simulink library "Collector_EN12975_FlatPlate_CONF"  (R2016b)
settings: Solver=ode45  StartTime=0.0  StopTime=10.0  RelTol=1e-3  EnableMultiTasking=on
undefined symbols (not defined in the file): Acol, path_carnot, Qdot, THBin, THBout
libraries: carnot x2
settings Model: Creator=lena.frank  LastModifiedBy=drhf
settings DataIOCC: LimitDataPoints=on  SaveFormat=Array  SignalLoggingSaveFormat=ModelDataLogs
settings OptimizationCC: ExpressionDepthLimit=2147483647  LifeSpan=inf
settings DebuggingCC: UnderspecifiedInitializationDetection=Classic  MergeDetectMultiDrivingBlocksExec=none  SolverPrmCheckMsg=warning  FcnCallInpInsideContextMsg=warning  StateNameClashWarn=warning  SFUnexpectedBacktrackingDiag=warning  SFNoUnconditionalDefaultTransitionDiag=warning  SFExecutionAtInitializationDiag=none
settings HardwareCC: ProdBitPerPointer=32  ProdBitPerSizeT=32  ProdBitPerPtrDiffT=32  ProdLargestAtomicFloat=None  ProdIntDivRoundTo=Undefined  ProdEndianess=Unspecified  ProdWordSize=32  ProdHWDeviceType=32-bit Generic
settings ModelReferenceCC: PropagateSignalLabelsOutOfModel=off
settings GRTTargetCC: TargetLangStandard=C89/C90 (ANSI)  GeneratePreprocessorConditionals=Disable all  CombineOutputUpdateFcns=off  GRTInterface=on
settings ConfigComp: CovMetricSettings=dw  CovHtmlReporting=on  CovSaveCumulativeToWorkspaceVar=on  CovSaveSingleToWorkspaceVar=on  CovExternalEMLEnable=off

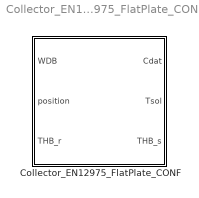
== system Collector_EN12975_FlatPlate_CONF ==
  Collector_EN12975_FlatPlate_CONF : Subsystem  mask(configurated Flat Plate Solar Thermal Collector){tini=20, Ncollector=2, PathName=fullfile(path_carnot('libsl'), 'Source','Solar_Thermal','Collector_EN12975_FlatPlate_CONF','parameter_set'), FileName='DefaultCollectorFlatPlate.mat', userPath=off, userParam=off, acol=2.5, len=2.3, fta=0.75, c1=3.5, c2=0.01, c3=0, c4=0, c5=7000, c6=0, b0=0.1, Kd=0.92, dplin=10, dpqua=10, SensorTimeConstant=10}
      mask prompts: tini "initial temperature [°C]"; Ncollector "Number of collectors in parallel"; PathName "Path"; FileName "Parameter set"; userPath "Edit path and name of parameter set"; userParam "User defined parameters"; acol "A : collector surface  [m²]"; len "length between inlet and outlet [m]"; fta "F'(TauAlfa)"; c1 "c1 : heat loss coefficient at (Tm-Ta)=0  [W/(m²*K)]"; c2 "c2: temperature dependence of the heat loss coefficient [W/(m*K)²]"; c3 "c3 : wind speed dependence of the heat loss coefficient [J/(m³K)]"; c4 "c4 : sky temperature dependence of the heat loss coefficient [W/(m²K)]"; c5 "c5 : effective thermal capacity [J/(m²K)]"; c6 "c6 : wind dependence of conversion factor [s/m]"; b0 "b0 : constant for the calculation of the incident angle modifier (direct radiation)"; Kd "Kd : Incidence angle modifier diffuse radiation"; dplin "linear pressure drop in Pa/(kg/s)"; dpqua "quadratic pressure drop in Pa/(kg/s)²"; SensorTimeConstant "time constant of sensor [s]"
      mask help:
      | Dynamic 1-node collector model according to EN 12975 standard using the b0 model for flat plate collector optics.
      | This block uses predefined parameter sets.
      mask init:
      | % callback to set parameters of model
      | [ok, param] = CarnotCallbacks_CollectorEN12975FlatPlateConf('SetParameters',gcbh,PathName,FileName);
      mask Help: web(fullfile(path_carnot('help'),'collector_en12975.html'),'-helpbrowser')
      mask TypeOptions tini: Collector_EN12975_FlatPlate/tini | T_Sensor1/t0
      mask TypeOptions Ncollector: Ncollector/Value
      mask Callback userPath: [ok, param] = CarnotCallbacks_CollectorEN12975FlatPlateConf('UserEdit',gcbh);
      mask Callback userParam: [ok, param] = CarnotCallbacks_CollectorEN12975FlatPlateConf('UserEdit',gcbh);
      mask TypeOptions acol: Collector_EN12975_FlatPlate/acol
      mask TypeOptions len: Collector_EN12975_FlatPlate/len
      mask TypeOptions fta: Collector_EN12975_FlatPlate/fta
      mask TypeOptions c1: Collector_EN12975_FlatPlate/c1
      mask TypeOptions c2: Collector_EN12975_FlatPlate/c2
      mask TypeOptions c3: Collector_EN12975_FlatPlate/c3
      mask TypeOptions c4: Collector_EN12975_FlatPlate/c4
      mask TypeOptions c5: Collector_EN12975_FlatPlate/c5
      mask TypeOptions c6: Collector_EN12975_FlatPlate/c6
      mask TypeOptions b0: Collector_EN12975_FlatPlate/b0
      mask TypeOptions Kd: Collector_EN12975_FlatPlate/Kd
      mask TypeOptions dplin: Collector_EN12975_FlatPlate/lin
      mask TypeOptions dpqua: Collector_EN12975_FlatPlate/qua
      mask TypeOptions SensorTimeConstant: T_Sensor1/tc
      mask DialogControl Control3 Prompt: Carnot public data
      mask DialogControl Control3 Callback: [ok, file] = CarnotCallbacks_CollectorEN12975FlatPlateConf('GetFilename',gcbh,'public');
      mask DialogControl Control4 Prompt: Carnot internal data
      mask DialogControl Control4 Callback: [ok, file] = CarnotCallbacks_CollectorEN12975FlatPlateConf('GetFilename',gcbh,'internal');
      mask DialogControl Control5 Prompt: Selected path
      mask DialogControl Control5 Callback: [ok, file] = CarnotCallbacks_CollectorEN12975FlatPlateConf('GetFilename',gcbh,'selected');
      mask DialogControl Control6 Prompt: Save in Carnot internal data
      mask DialogControl Control6 Callback: [ok, param] = CarnotCallbacks_CollectorEN12975FlatPlateConf('SaveFilename',gcbh,'internal','FPC');
      mask DialogControl Control7 Prompt: Save in selected path
      mask DialogControl Control7 Callback: [ok, param] = CarnotCallbacks_CollectorEN12975FlatPlateConf('SaveFilename',gcbh,'selected','FPC');
      mask Display:
      | % user defined picture file
      | picfile = fullfile(path_carnot('intlibsl'), ...
      |     'Source','Solar_Thermal','Collector_EN12975_FlatPlate_CONF','parameter_set', ...
      |     'Collector_CONF.jpg');
      | 
      | pic = false;
      | 
      | % show internal picture if defined
      | if ~BlockIsInCarnotLibrary    % if not located in library any more
      |     if exist(picfile)
      |         image(imread(picfile), [0.2, 0, 0.6, 1])
      |         set_param(gcb, 'BackgroundColor', 'White')
      |         pic = true;
      |     end
      | end
      | 
      | if ~pic % show public picture
      |     set_param(gcb, 'BackgroundColor', 'Yellow')
      |     disp('solar thermal\ncollector\nEN 12975\nB0-Optics')
      | end
      | 
      | % Show port labels: same as port labels in the subsystem,
      | % but display with a picture covers the text. Have to reprint it.
      | % port_label('input',1,'WDB')
      | % port_label('input',2,'position')
      | % port_label('input',3,'THB_r')
      | % port_label('output',1,'Cdat')
      | % port_label('output',2,'Tsol')
      | % port_label('output',3,'THB_s')

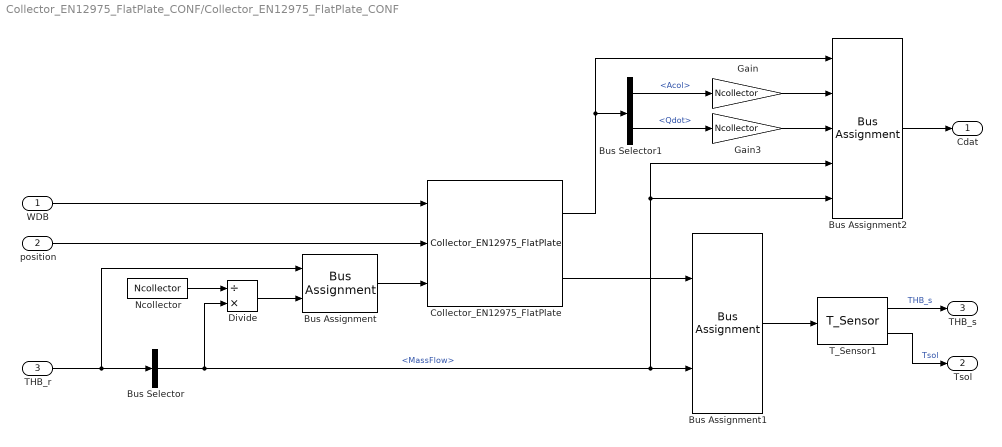
== system Collector_EN12975_FlatPlate_CONF/Collector_EN12975_FlatPlate_CONF ==
  WDB : Inport
  position : Inport  Port=2
  THB_r : Inport  Port=3
  Bus Assignment : BusAssignment  AssignedSignals=MassFlow
  Bus Assignment1 : BusAssignment  AssignedSignals=MassFlow
  Bus Assignment2 : BusAssignment  AssignedSignals=Acol,Qdot,THBin.MassFlow,THBout.MassFlow
  Bus Selector : BusSelector  OutputSignals=MassFlow
  Bus Selector1 : BusSelector  OutputSignals=Acol,Qdot
  Collector_EN12975_FlatPlate : carnot/Source/Solar_Thermal/Collector_EN12975_FlatPlate  acol=acol  len=len  fta=fta  c1=c1  c2=c2  c3=c3  c4=c4  c5=c5  c6=c6  b0=b0  Kd=Kd  lin=dplin  qua=dpqua  tini=tini
  Divide : Product  Inputs=/*
  Gain : Gain  Gain=Ncollector
  Gain3 : Gain  Gain=Ncollector
  Ncollector : Constant  Value=Ncollector
  T_Sensor1 : carnot/Control/T_Sensor  tc=SensorTimeConstant  t0=tini
  Cdat : Outport
  Tsol : Outport  Port=2
  THB_s : Outport  Port=3
  wires:
  T_Sensor1/1 -> THB_s/1  "THB_s"
  T_Sensor1/2 -> Tsol/1  "Tsol"
  Bus Assignment2/1 -> Cdat/1
  Gain3/1 -> Bus Assignment2/3
  Gain/1 -> Bus Assignment2/2
  Bus Selector1/2 -> Gain3/1  "<Qdot>"
  Bus Selector1/1 -> Gain/1  "<Acol>"
  Divide/1 -> Bus Assignment/2
  Ncollector/1 -> Divide/1
  Bus Selector/1 -> Bus Assignment1/2, Bus Assignment2/4, Bus Assignment2/5, Divide/2  "<MassFlow>"
  Bus Assignment1/1 -> T_Sensor1/1
  Bus Assignment/1 -> Collector_EN12975_FlatPlate/3
  Collector_EN12975_FlatPlate/1 -> Bus Selector1/1, Bus Assignment2/1
  THB_r/1 -> Bus Selector/1, Bus Assignment/1
  position/1 -> Collector_EN12975_FlatPlate/2
  WDB/1 -> Collector_EN12975_FlatPlate/1
  Collector_EN12975_FlatPlate/2 -> Bus Assignment1/1
